simulink model "singleRotor_speedCTRL_dynInflow_PittPeters"  (R2022b)
settings: Solver=ode45  StartTime=0.0  StopTime=55  RelTol=1e-4  EnableMultiTasking=on
InitFcn:
  | dir = pwd; %model directory
  | 
  | %go to look up tables
  | cd('../Look Up Tables/') %look up table directory
  | 
  | % %Ct, Cp, and theta of rotor from BEMT (for comparison)
  | load("BEMT-3.mat");
  | 
  | %Rotor and Pitt-Peters model parameters (M,L,k)
  | load("PP-2.mat");
  | k = model.k; %mass flow correction
  | 
  | %go back to model directory
  | cd(pwd);
  | 
  | %Hide scope plots
  | HidHandles = get(0,'ShowHiddenHandles');
  | set(0,'ShowHiddenHandles','On');
  | AllScopeHandles = findobj(0,'Type','Figure','Tag','SIMULINK_SIMSCOPE_FIGURE');
  | close(AllScopeHandles);
  | set(0,'ShowHiddenHandles',HidHandles);
  | 
  | %Working Directory
  | directory = pwd;
  | 
  | %Atmospheric Properties
  | rho_air = 1.225;  % air density in kg/m^3
  | mu = 1.803e-5; % dynamic viscosity [N-s/m^2]
  | 
  | Vbus = 300;  % Actual bus voltage (volts) that will be applied
  | % Emrax 208
  | R = .0122;  %  resistance, ohms, line-line at room temp
  | L = 125*10^-6;  %  inductance line-line at commutation frequency, henries
  | t_elec = L/R;
  | 
  | Irotor = 256/100^2;  %  kg*m^2 -- From Emrax data sheet
  | Kt_motor = .8005;  %  N*m/Arms (measured from 05/25/2023 test_c data)
  | Ke_motor = .0487*sqrt(2)*60/(2*pi);  %  Vpk/rad/sec
  | Ke = .0487*sqrt(2)*60/(2*pi);   %radians/sec
  | 
  | CurrentSenseMax = 250;  %  Max current sense from controller code
  | BASE_CURRENT = 125;   %  Max current in amps corresponding to normalized control loop current = 1
  | LOOP_FREQUENCY = 35;     % orig: 35 in kHz
  | T_LOOP = .001/LOOP_FREQUENCY;
  | pwm_loop_prescalar = 1;  %Presacalar how many PWM cycles for one current loop execution
  | T_PWM = T_LOOP/pwm_loop_prescalar;  %  Current loop prescaler on PWM is 1 for Uber
  | POLES = 20;
  | BASE_FREQ = 1200; %POLES/2*1300/60;  %  1300 rpm
  | BaseSpeed     = BASE_FREQ*(60.0/(POLES/2.0));
  | 
  | % current loop
  | alpha = 250*2*pi;         % current loop bandwidth
  | 
  | omega = 0;               % omega for de-coupling integrator
  | 
  | % no-load current fit (i0 = a1*omega^2 + a2) [Apk]
  | i_a1 = 8.98e-5;
  | i_a2 = 2.51;
  | 
  | % Current loop
  | %          Motor_Params.ILOOP_BW = (2*PI*1000.0);
  | %        Motor_Params.id_KP = Motor_Params.ILOOP_BW*Motor_Params.StatorInductance;
  | %      Motor_Params.id_KI = Motor_Params.ILOOP_BW*Motor_Params.StatorResistance;
  | %      Motor_Params.iq_KP = Motor_Params.ILOOP_BW*Motor_Params.StatorInductance;
  | %     Motor_Params.iq_KI = Motor_Params.ILOOP_BW*Motor_Params.StatorResistance;
  | I_Kp = alpha*L*1;
  | I_Ki = alpha*R/I_Kp*T_LOOP;
  | %I_Ki = alpha*R*0;
  | 
  | % Speed loop
  | %------------%
  | %NOTES
  | %Originial Kp = 3.0 and Ki = 0.15*Tspeedloop*1.5
  | %Kp = 4.75 and Ki = 2.5e-4 led to only ~1-2s response time indep. of slew rate
  | %Kp = 15 and Ki = 2.1*Tspeedloop*1.5 led to 0.4s response time with slight overshoot
  | %------------%
  | SpeedLoopPrescale = 5;
  | Tspeedloop = T_LOOP*SpeedLoopPrescale;
  | % PID_spd_Kp = 18;   % From Uber code (ORIGINIAL: 3)
  | % PID_spd_Ki = 1*Tspeedloop;   % From Uber code (ORIGINAL: 0.15*Tspeedloop*2)
  | PID_spd_Kp = 31;   % From Uber code (ORIGINIAL: 3)
  | PID_spd_Ki = .128*Tspeedloop;   % From Uber code (ORIGINAL: 0.15*Tspeedloop*2)
  | 
  | Ramp_sec = 1250;    %  Ramp slew rate limiter, [rpm/s]
  | 
  | % Position loop
  | speedErrorPEngage = .003; % Speed error max for position loop to enable
  | % Code has .001 for PEngage, trying something diff here
  | PID_pos_Kp = 3.5; %on MC40: 2.5 (changed on 23 OCT 2021)
  | PID_pos_Ki = .00001; % orig: 0.00003
  | PID_pos_Kd = 8000; % on MC40: 8000
  | 
  | PID_pos_error_sat = .3;  % ORIG = 0.3 Maximum error saturated into position PID (in simulink, not C right now)
  | PID_pos_sat = .25;  %  From code, based on DC bus limit (orig: .25)
  | PID_pos_C1 = .999; % ORIG = 1 Position loop D bandlimit filter
  | PID_pos_C2 = .001;  % ORIG = 0 Position loop D bandlimit filter
  | 
  | 
  | % transfer function of speed estimator is K1*K3*z/(z-K2)
  | %  Pole is at z = K2
  | % z = exp(-sT)
  | f_estpole = 35000;  %orig: 35000
  | K1 = 1/(BASE_FREQ*T_LOOP);   %  Divide by base freq to convert from elec delta-normalized-angle/cycle to [0,1] normalized speed
  |      %  K1 converts delta angle estimate over a loop period to a [0,1] speed estimate
  | K2 = exp(-f_estpole*2*pi*T_LOOP);
  | K3 = 1 - K2;  % Set to make filter have unity gain at 0 frequency (z = 1)
  | 
  | %Rotor properties
  | %{---------------- COAX ------------------------
  | % d_prop = 2.216;   %  diameter propeller [m] 2.032 (coax) 2.216 (stacked)
  | % R_c = d_prop/2*.19; % root cutout [m]
  | % c = 0.08; %chord [m]
  | % nb = 2; %number of blades
  | % sigma = nb*c/pi/(d_prop/2);
  | % I_emp = rotor_params.I_rotor; %from dynamic RPM testing (230313 test k and l)
  | % I_emp = 0.248; %CAD inertia
  | % I_emp = 0.40481; %from dynamic RPM testing (230313 test k and l)
  | % GR = 1.2;
  | % kappa = rotor_params.kappa;
  | % dr = rotor_params.dr;
  | % Cp0 = 5.908e-5; %profile power coefficient (230314 steady)
  | % Cp0 = 6.167e-05; %profile power (230525_test_c steady -- stacked rotor)
  | %-------------------------------------------------
  | %}
  | 
  | %{---------------- UBER ------------------------
  | d_prop = 2*rotor_params.R;   %  diameter propeller [m] 2.032 (coax) 2.216 (stacked)
  | R_c = rotor_params.R_cutout; % root cutout [m]
  | c = rotor_params.c; %chord [m]
  | nb = rotor_params.Nb; %number of blades
  | sigma = nb*c/pi/(d_prop/2);
  | I_emp = rotor_params.I_rotor; %from dynamic RPM testing (230525 test a) [kg*m2]
  | I_m = 0.2717; %from dynamic RPM testing (230525 test a) [kg*m2]
  | % I_m = 2*0.3662; %4-bladed comparison motor inerita. 2X the motor inertia from 231113 testing
  | GR = 1.2;
  | kappa = rotor_params.kappa;
  | dr = rotor_params.dr;
  | Cp0 = rotor_params.Cp0; %profile power (230525_test_c steady -- stacked rotor)
  | %-------------------------------------------------
  | %}
  | 
  | 
  | InitialRPM = 950*GR;
  | omegamech = InitialRPM/60*2*pi;  %  Used to preload Q current voltage integrator
  | 
  | % Serial Message frequency (messages per second)
  | MsgFreq = 1000;
  | 
  | cd(dir);
values from neighbouring files (symbols this model uses):
  Ct = [0 8.42066058624e-05 0.000168413211725 0.000252619817587 0.000348569118235 0.000435711397794 0.000522853677352 0.000609995956911 0.00069713823647 0.000784280516029 0.000871422795587 0.000958565075146 ... (150 elements, 1x150)]    [BEMT-1.mat]    (also in BEMT-2.mat = [-0.000241284312952 -0.00019885713846 -0.000156429963968 -0.; BEMT-3.mat = [-0.000252881464423 -0.00020500571035 -0.00015767832519 -0.0; BEMT-PF-Isolated-1.mat = [-0.000124730397385 6.78902114512e-07 0.000152796242494 0.00; BEMT-PF-Isolated-2.mat = [-0.000124743531158 6.68801957239e-07 0.000152879013625 0.00)
  model =     [DynInflow-1.mat]    (also in PP-1.mat; PP-2.mat; PP-3.mat)
  rotor_params =     [DynInflow-1.mat]    (also in PP-1.mat; PP-2.mat; PP-3.mat)
  theta = [-1.24244156171 -0.730247869575 -0.489791195362 -0.291308360013 -0.0904887039498 0.0775201787218 0.236938510902 0.389966557012 0.537998944025 0.680941129328 0.820002111662 0.955737387113 ... (150 elements, 1x150)]    [BEMT-1.mat]    (also in BEMT-2.mat = [-2.67472972391 -2.52181622329 -2.35655527709 -2.17339529035; BEMT-3.mat = [-2.61565298703 -2.45920727031 -2.29202818901 -2.11251263407; BEMT-PF-Isolated-1.mat = [-2 -1 0 1 2 3 4 5 6 7 8 9 ... (16 elements, 1x16)]; BEMT-PF-Isolated-2.mat = [-2 -1 0 1 2 3 4 5 6 7 8 9 ... (16 elements, 1x16)])
undefined symbols (not defined in the file or in its folder): DiscIntNeverNeededParam
libraries: eeGeneralControl x1
settings Model: ModifiedHistory=4/7/2020 Adding in voltage saturation to mag 1 before SVGEN  Creator=mricci  LastModifiedBy=msa2925
settings SolverCC: AlgebraicLoopSolver=TrustRegion
settings DataIOCC: LimitDataPoints=on  SaveFormat=Array  SignalLoggingSaveFormat=ModelDataLogs  ReturnWorkspaceOutputs=off
settings OptimizationCC: ExpressionDepthLimit=2147483647  InitFltsAndDblsToZero=on  LifeSpan=inf
settings DebuggingCC: UnderspecifiedInitializationDetection=Classic  MergeDetectMultiDrivingBlocksExec=none  SolverPrmCheckMsg=warning  FcnCallInpInsideContextMsg=warning  UnconnectedInputMsg=warning  UnconnectedOutputMsg=warning  UnconnectedLineMsg=warning  StateNameClashWarn=warning  SFUnexpectedBacktrackingDiag=warning  SFNoUnconditionalDefaultTransitionDiag=warning  SFExecutionAtInitializationDiag=none  SFMachineParentedDataDiag=warning  ArithmeticOperatorsInVariantConditions=warning
settings HardwareCC: ProdBitPerPointer=32  ProdBitPerSizeT=32  ProdBitPerPtrDiffT=32  ProdLargestAtomicFloat=None  ProdIntDivRoundTo=Undefined  ProdEndianess=Unspecified  ProdWordSize=32  ProdHWDeviceType=32-bit Generic
settings ModelReferenceCC: EnableRefExpFcnMdlSchedulingChecks=on  PropagateSignalLabelsOutOfModel=off
settings RTWCC: DLArmComputeVersion=19.05
settings CodeAppCC: StateflowObjectComments=on
settings GRTTargetCC: TargetLangStandard=C89/C90 (ANSI)  CombineOutputUpdateFcns=off  GRTInterface=on
settings ConfigComp: CovMetricSettings=dw  CovSaveCumulativeToWorkspaceVar=on  CovSaveSingleToWorkspaceVar=on

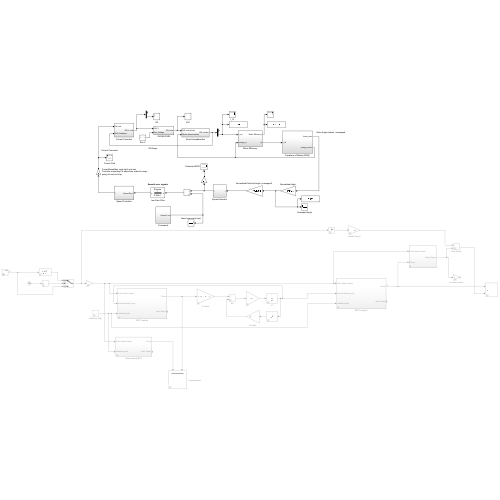
[thumbnail: Simulink's stored preview of the top-level diagram]
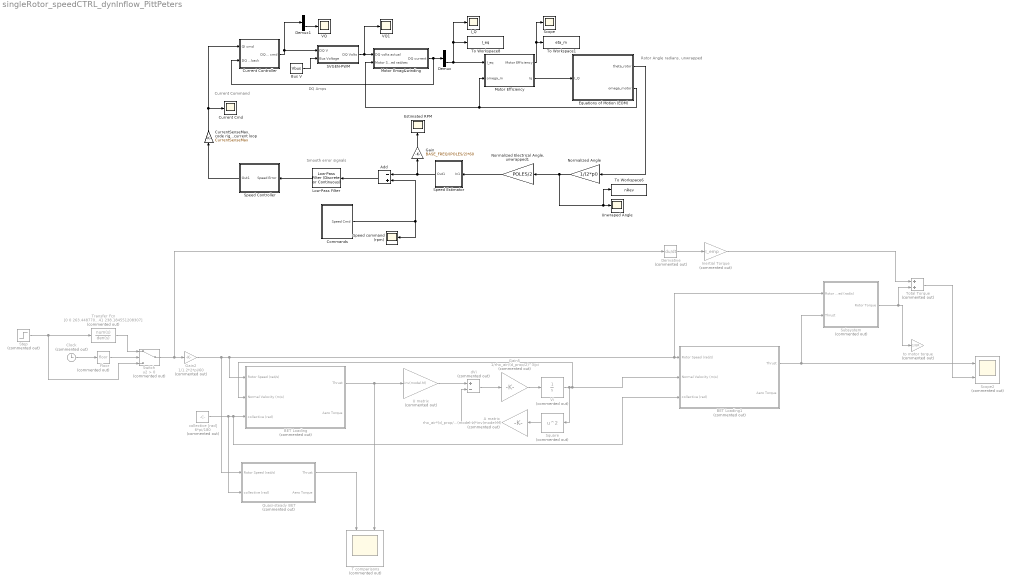
== system singleRotor_speedCTRL_dynInflow_PittPeters ==
  note: Smooth error signals
  note: Current Command
  note: Rotor Angle radians, unwrapped
  note: DQ Amps
  A matrix : Gain  Commented=on  Gain=rho_air*(d_prop/2)^2*pi*k*inv(model.L)*inv(model.M)
  Add : Sum  Inputs=-+
  BET Loading : Subsystem  Commented=on
  BET Loading1 : Subsystem  Commented=on
  Bus V : Constant  Value=Vbus
  Clock : Clock  Commented=on
  Commands : Subsystem
  Current Cmd : Scope
  Current Controller : Subsystem
  "CurrentSenseMax, code right now has Controller outputting PU amps then scaled to amps going into current loop" : Gain  Gain=CurrentSenseMax
  Demux : Demux  Outputs=2
  Demux1 : Demux  Outputs=2
  Derivative : Derivative  Commented=on
  Equations of Motion (EOM) : Subsystem
  Estimated RPM : Scope
  Floor : Rounding  Commented=on
  Gain : Gain  Gain=BASE_FREQ/(POLES/2)*60
  Gain2 : Gain  Commented=on  Gain=1/1.2*2*pi/60
  Gain5 : Gain  Commented=on  Gain=1/rho_air/(d_prop/2)^3/pi
  I_Q : Scope
  Inertial Torque : Gain  Commented=on  Gain=I_emp
  Low-Pass Filter : eeGeneralControl/Low-Pass Filter (Discrete or Continuous)  K=1  T=3e-2  B=inf  A=-inf  init_option=Inherited from block input  x0=0  Ts=-1
  Motor Efficiency : Subsystem
  Motor Emag&winding : Subsystem
  Normalized Angle : Gain  Gain=1/(2*pi)
  "Normalized Electrical Angle, unwrapped1" : Gain  Gain=POLES/2
  Quasi-steady BET : Subsystem  Commented=on
  SVGEN-PWM : Subsystem
  Scope : Scope
  Scope2 : Scope  Commented=on  NumInputPorts=2
  Speed Controller : Subsystem
  Speed Estimator : Subsystem
  Speed command (rpm) : Scope
  Square : Math  Commented=on  Operator=square
  Step : Step  Commented=on  Time=50  Before=InitialRPM  After=InitialRPM+30*GR  SampleTime=0
  Subsystem : Subsystem  Commented=on
  Switch : Switch  Commented=on  Criteria=u2 > Threshold  SaturateOnIntegerOverflow=off  InputSameDT=off
  T comparisons : Scope  Commented=on  NumInputPorts=2
  To Workspace1 : ToWorkspace  VariableName=eta_m  SaveFormat=Timeseries  SampleTime=-1
  To Workspace6 : ToWorkspace  VariableName=nRev  SaveFormat=Timeseries  SampleTime=-1
  To Workspace8 : ToWorkspace  VariableName=I_eq  SaveFormat=Timeseries  SampleTime=-1
  Total Torque : Sum  Commented=on
  Transfer Fcn : TransferFcn  Commented=on  Numerator="[0\t0\t263.448770344578]"  Denominator="[1\t17.1002833911441\t238.184551208307]"
  U matrix : Gain  Commented=on  Gain=inv(model.M)
  Unwraped Angle : Scope
  VQ : Scope
  VQ1 : Scope
  Vi : Integrator  Commented=on  InitialCondition=5.9
  collective [rad] : Constant  Commented=on  Value=6*pi/180
  dVi : Sum  Commented=on  Inputs=+-
  to motor torque : Gain  Commented=on  Gain=1/GR
  wires:
  Speed Estimator/1(Out1) -> Add/1, Gain/1
  Gain/1 -> Estimated RPM/1
  Add/1 -> Low-Pass Filter/1
  "CurrentSenseMax, code right now has Controller outputting PU amps then scaled to amps going into current loop"/1 -> Current Controller/1(QI cmd), Current Cmd/1
  Equations of Motion (EOM)/2(omega_motor) -> Motor Efficiency/2(omega_m), Motor Emag&winding/2(Motor Speed rad/sec)
  Motor Emag&winding/1(DQ current) -> Current Controller/2(DQ I feedback), Demux/1
  Demux/2 -> Motor Efficiency/1(I_eq), To Workspace8/1, I_Q/1
  Equations of Motion (EOM)/1(theta_rotor) -> Normalized Angle/1
  Normalized Angle/1 -> "Normalized Electrical Angle, unwrapped1"/1, To Workspace6/1, Unwraped Angle/1
  "Normalized Electrical Angle, unwrapped1"/1 -> Speed Estimator/1(In1)
  Commands/1(Speed Cmd) -> Add/2, Speed command (rpm)/1
  Speed Controller/1(Out1) -> "CurrentSenseMax, code right now has Controller outputting PU amps then scaled to amps going into current loop"/1
  Demux1/2 -> VQ/1
  Low-Pass Filter/1 -> Speed Controller/1(Speed Error)
  SVGEN-PWM/1(DQ Volts) -> VQ1/1, Motor Emag&winding/1(DQ volts actual)
  Bus V/1 -> SVGEN-PWM/2(Bus Voltage)
  Current Controller/1(DQ V cmd) -> SVGEN-PWM/1(DQ V), Demux1/1
  Motor Efficiency/2(Iq) -> Equations of Motion (EOM)/1(I_Q)
  Motor Efficiency/1(Motor Efficiency) -> Scope/1, To Workspace1/1
  Gain2/1 -> Subsystem/1(Rotor Speed (rad/s)), BET Loading1/1(Rotor Speed (rad/s)), BET Loading/1(Rotor Speed (rad/s)), Quasi-steady BET/1(Rotor Speed (rad/s))
  A matrix/1 -> dVi/2
  Quasi-steady BET/1(Thrust) -> T comparisons/2
  collective [rad]/1 -> BET Loading/3(collective (rad)), BET Loading1/3(collective (rad)), Quasi-steady BET/2(collective (rad))
  Square/1 -> A matrix/1
  U matrix/1 -> dVi/1
  Gain5/1 -> Vi/1
  BET Loading/1(Thrust) -> T comparisons/1, U matrix/1
  dVi/1 -> Gain5/1
  Vi/1 -> BET Loading1/2(Normal Velocity (m/s)), BET Loading/2(Normal Velocity (m/s)), Square/1
  BET Loading1/1(Thrust) -> Subsystem/2(Thrust), Scope2/1
  Switch/1 -> Derivative/1, Gain2/1
  Transfer Fcn/1 -> Switch/1
  Step/1 -> Transfer Fcn/1, Switch/3
  Floor/1 -> Switch/2
  Clock/1 -> Floor/1
  Subsystem/1(Rotor Torque) -> Total Torque/2, to motor torque/1
  Derivative/1 -> Inertial Torque/1
  Total Torque/1 -> Scope2/2
  Inertial Torque/1 -> Total Torque/1

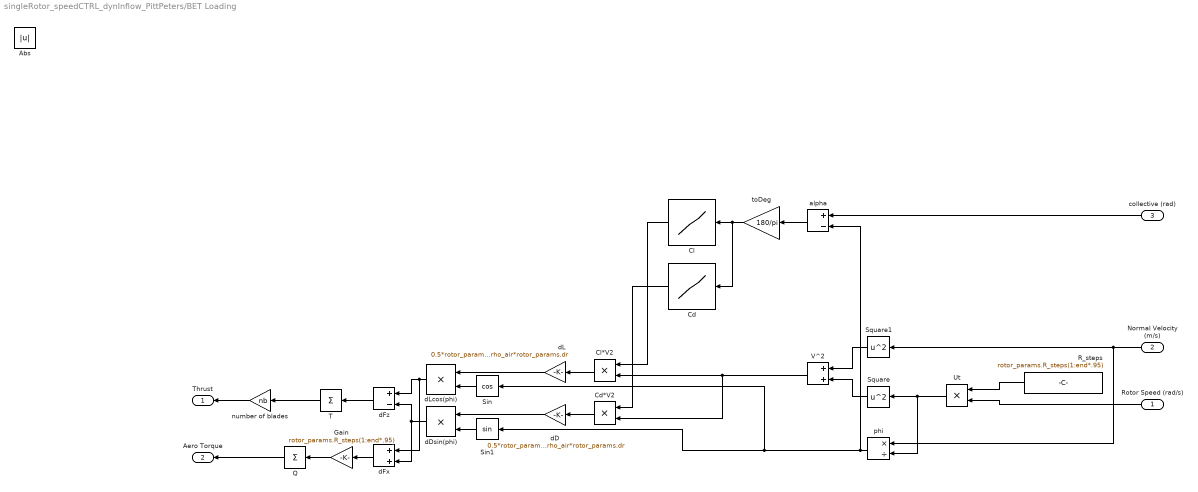
== system singleRotor_speedCTRL_dynInflow_PittPeters/BET Loading ==
  Rotor Speed (rad/s) : Inport
  Normal Velocity (m/s) : Inport  Port=2
  collective (rad) : Inport  Port=3
  Abs : Abs  SaturateOnIntegerOverflow=off
  Cd : Lookup_n-D  NumberOfTableDimensions=1  BreakpointsForDimension1=rotor_params.AoA  BreakpointsForDimension2=[1:3]  Table=rotor_params.Cd  InternalRulePriority=Speed  RndMeth=Simplest
  Cd*V2 : Product
  Cl : Lookup_n-D  NumberOfTableDimensions=1  BreakpointsForDimension1=rotor_params.AoA  BreakpointsForDimension2=[1:3]  Table=rotor_params.Cl  UseLastTableValue=on  InternalRulePriority=Speed  RndMeth=Simplest
  Cl*V2 : Product
  Gain : Gain  Gain=rotor_params.R_steps(1:end*.95)
  Q : Sum  Inputs=+
  R_steps : Constant  Value=rotor_params.R_steps(1:end*.95)
  Sin : Trigonometry  Operator=cos
  Sin1 : Trigonometry
  Square : Math  Operator=square
  Square1 : Math  Operator=square
  T : Sum  Inputs=+
  Ut : Product
  V^2 : Sum
  alpha : Sum  Inputs=+-
  dD : Gain  Gain=0.5*rotor_params.c*rho_air*rotor_params.dr
  dDsin(phi) : Product
  dFx : Sum
  dFz : Sum  Inputs=+-
  dL : Gain  Gain=0.5*rotor_params.c*rho_air*rotor_params.dr
  dLcos(phi) : Product
  number of blades : Gain  Gain=nb
  phi : Product  Inputs=*/
  toDeg : Gain  Gain=180/pi
  Thrust : Outport
  Aero Torque : Outport  Port=2
  wires:
  T/1 -> number of blades/1
  alpha/1 -> toDeg/1
  Normal Velocity (m/s)/1 -> phi/1, Square1/1
  Rotor Speed (rad/s)/1 -> Ut/2
  phi/1 -> Sin/1, Sin1/1, alpha/2
  collective (rad)/1 -> alpha/1
  Square/1 -> V^2/2
  Square1/1 -> V^2/1
  Ut/1 -> phi/2, Square/1
  V^2/1 -> Cl*V2/2, Cd*V2/2
  R_steps/1 -> Ut/1
  Cl*V2/1 -> dL/1
  Cd*V2/1 -> dD/1
  Sin/1 -> dLcos(phi)/2
  dL/1 -> dLcos(phi)/1
  dD/1 -> dDsin(phi)/1
  Sin1/1 -> dDsin(phi)/2
  dLcos(phi)/1 -> dFx/1, dFz/1
  dDsin(phi)/1 -> dFx/2, dFz/2
  dFz/1 -> T/1
  number of blades/1 -> Thrust/1
  toDeg/1 -> Cl/1, Cd/1
  Cd/1 -> Cd*V2/1
  Q/1 -> Aero Torque/1
  dFx/1 -> Gain/1
  Gain/1 -> Q/1
  Cl/1 -> Cl*V2/1

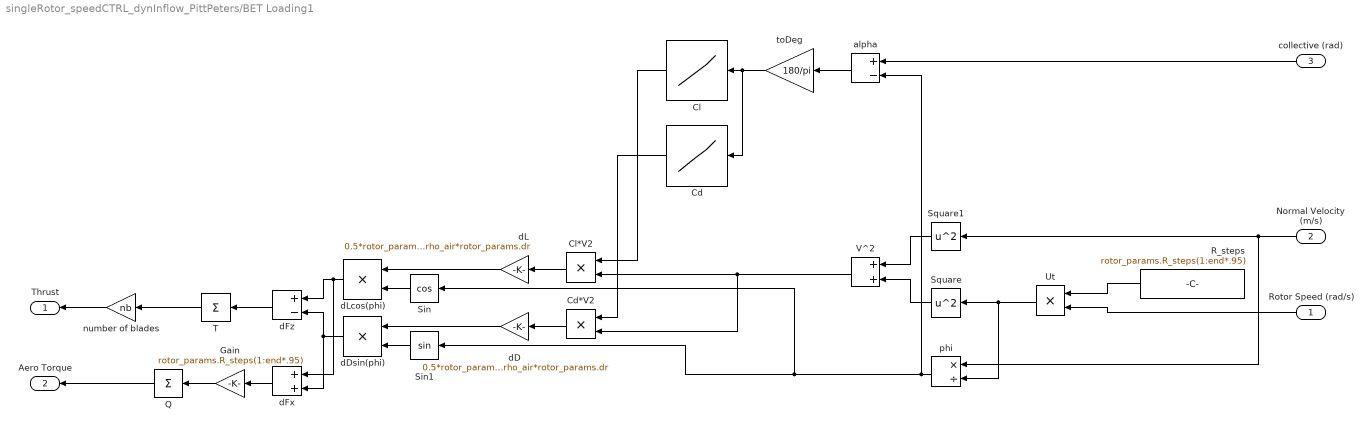
== system singleRotor_speedCTRL_dynInflow_PittPeters/BET Loading1 ==
  Rotor Speed (rad/s) : Inport
  Normal Velocity (m/s) : Inport  Port=2
  collective (rad) : Inport  Port=3
  Cd : Lookup_n-D  NumberOfTableDimensions=1  BreakpointsForDimension1=rotor_params.AoA  BreakpointsForDimension2=[1:3]  Table=rotor_params.Cd  InternalRulePriority=Speed  RndMeth=Simplest
  Cd*V2 : Product
  Cl : Lookup_n-D  NumberOfTableDimensions=1  BreakpointsForDimension1=rotor_params.AoA  BreakpointsForDimension2=[1:3]  Table=rotor_params.Cl  UseLastTableValue=on  InternalRulePriority=Speed  RndMeth=Simplest
  Cl*V2 : Product
  Gain : Gain  Gain=rotor_params.R_steps(1:end*.95)
  Q : Sum  Inputs=+
  R_steps : Constant  Value=rotor_params.R_steps(1:end*.95)
  Sin : Trigonometry  Operator=cos
  Sin1 : Trigonometry
  Square : Math  Operator=square
  Square1 : Math  Operator=square
  T : Sum  Inputs=+
  Ut : Product
  V^2 : Sum
  alpha : Sum  Inputs=+-
  dD : Gain  Gain=0.5*rotor_params.c*rho_air*rotor_params.dr
  dDsin(phi) : Product
  dFx : Sum
  dFz : Sum  Inputs=+-
  dL : Gain  Gain=0.5*rotor_params.c*rho_air*rotor_params.dr
  dLcos(phi) : Product
  number of blades : Gain  Gain=nb
  phi : Product  Inputs=*/
  toDeg : Gain  Gain=180/pi
  Thrust : Outport
  Aero Torque : Outport  Port=2
  wires:
  T/1 -> number of blades/1
  alpha/1 -> toDeg/1
  Normal Velocity (m/s)/1 -> phi/1, Square1/1
  Rotor Speed (rad/s)/1 -> Ut/2
  phi/1 -> Sin/1, Sin1/1, alpha/2
  collective (rad)/1 -> alpha/1
  Square/1 -> V^2/2
  Square1/1 -> V^2/1
  Ut/1 -> phi/2, Square/1
  V^2/1 -> Cl*V2/2, Cd*V2/2
  R_steps/1 -> Ut/1
  Cl*V2/1 -> dL/1
  Cd*V2/1 -> dD/1
  Sin/1 -> dLcos(phi)/2
  dL/1 -> dLcos(phi)/1
  dD/1 -> dDsin(phi)/1
  Sin1/1 -> dDsin(phi)/2
  dLcos(phi)/1 -> dFx/1, dFz/1
  dDsin(phi)/1 -> dFx/2, dFz/2
  dFz/1 -> T/1
  number of blades/1 -> Thrust/1
  toDeg/1 -> Cd/1, Cl/1
  Cd/1 -> Cd*V2/1
  Q/1 -> Aero Torque/1
  dFx/1 -> Gain/1
  Gain/1 -> Q/1
  Cl/1 -> Cl*V2/1

== system singleRotor_speedCTRL_dynInflow_PittPeters/Commands ==
  "Normalized Speed [0,1] relative to \"base freq" : Gain  Gain=1/BaseSpeed
  Rate Limiter : RateLimiter  RisingSlewLimit=Ramp_sec  FallingSlewLimit=-Ramp_sec  SampleTimeMode=inherited  InitialCondition=InitialRPM/BaseSpeed
  Step : Step  Time=50  Before=InitialRPM  After=InitialRPM + 30*GR  SampleTime=0
  To Workspace5 : ToWorkspace  VariableName=Speed_cmd  SaveFormat=Timeseries  SampleTime=-1
  td : TransportDelay  DelayTime=.02
  Speed Cmd : Outport
  wires:
  "Normalized Speed [0,1] relative to \"base freq"/1 -> Speed Cmd/1
  Step/1 -> td/1, To Workspace5/1
  td/1 -> "Normalized Speed [0,1] relative to \"base freq"/1

== system singleRotor_speedCTRL_dynInflow_PittPeters/Current Controller ==
  note: Q current PI controller
  note: D current PI controller
  note: D Current Reference
  note: D Current Feedback
  note: Q Current Reference
  note: Discrete
      | time control
      | law
  QI cmd : Inport
  DQ I feedback : Inport  Port=2
  1/Ts gain DT integrator : DiscreteIntegrator  gainval=1/T_LOOP  InitialCondition=80  SampleTime=-1  LimitOutput=on  UpperSaturationLimit=Vbus*sqrt(3)  LowerSaturationLimit=-Vbus*sqrt(3)  ICPrevOutput=DiscIntNeverNeededParam  ICPrevScaledInput=DiscIntNeverNeededParam
  Constant : Constant  Value=0
  Demux : Demux  Outputs=2
  Gain : Gain  Gain=I_Kp
  Gain1 : Gain  Gain=I_Ki
  Gain2 : Gain  Gain=I_Kp
  Gain3 : Gain  Gain=I_Ki
  K=1/Ts DT itegrator : DiscreteIntegrator  gainval=1/T_LOOP  InitialCondition=-2  SampleTime=-1  LimitOutput=on  UpperSaturationLimit=Vbus*sqrt(3)  LowerSaturationLimit=-Vbus*sqrt(3)  ICPrevOutput=DiscIntNeverNeededParam  ICPrevScaledInput=DiscIntNeverNeededParam
  Mux1 : Mux  Inputs=2
  Sum : Sum  Inputs=|++
  Sum1 : Sum  Inputs=|++
  Sum2 : Sum  Inputs=|+-
  Sum3 : Sum  Inputs=|+-
  DQ V cmd : Outport
  wires:
  Mux1/1 -> DQ V cmd/1
  Constant/1 -> Sum2/1
  QI cmd/1 -> Sum3/1
  Sum/1 -> Mux1/1
  Sum1/1 -> Mux1/2
  DQ I feedback/1 -> Demux/1
  Demux/1 -> Sum2/2
  Demux/2 -> Sum3/2
  K=1/Ts DT itegrator/1 -> Sum/2
  Gain1/1 -> K=1/Ts DT itegrator/1
  Gain/1 -> Sum/1, Gain1/1
  Sum2/1 -> Gain/1
  Sum3/1 -> Gain2/1
  Gain2/1 -> Sum1/1, Gain3/1
  Gain3/1 -> 1/Ts gain DT integrator/1
  1/Ts gain DT integrator/1 -> Sum1/2

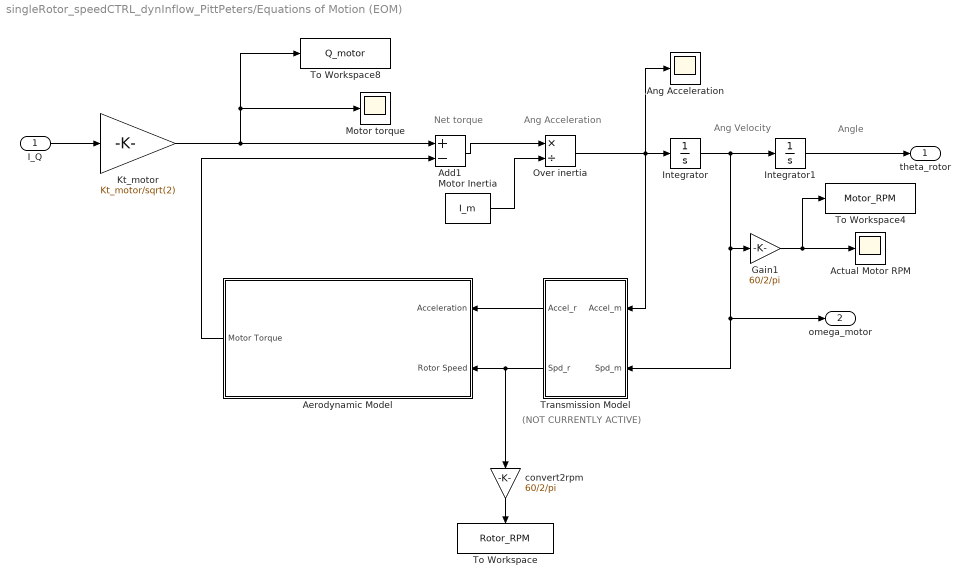
== system singleRotor_speedCTRL_dynInflow_PittPeters/Equations of Motion (EOM) ==
  note: (NOT CURRENTLY ACTIVE)
  note: Ang Acceleration
  note: Angle
  note: Ang Velocity
  note: Net torque
  I_Q : Inport
  Actual Motor RPM : Scope
  Add1 : Sum  Inputs=+-
  Aerodynamic Model : Subsystem
  Ang Acceleration : Scope
  Gain1 : Gain  Gain=60/2/pi
  Integrator : Integrator  InitialCondition=InitialRPM*2*pi/60
  Integrator1 : Integrator
  Kt_motor : Gain  Gain=Kt_motor/sqrt(2)
  Motor Inertia : Constant  Value=I_m
  Motor torque : Scope
  Over inertia : Product  Inputs=*/
  To Workspace : ToWorkspace  VariableName=Rotor_RPM  SaveFormat=Timeseries  SampleTime=-1
  To Workspace4 : ToWorkspace  VariableName=Motor_RPM  SaveFormat=Timeseries  SampleTime=-1
  To Workspace8 : ToWorkspace  VariableName=Q_motor  SaveFormat=Timeseries  SampleTime=-1
  Transmission Model : Subsystem
  convert2rpm : Gain  Gain=60/2/pi
  theta_rotor : Outport
  omega_motor : Outport  Port=2
  wires:
  I_Q/1 -> Kt_motor/1
  Integrator1/1 -> theta_rotor/1
  Add1/1 -> Over inertia/1
  Kt_motor/1 -> To Workspace8/1, Motor torque/1, Add1/1
  Gain1/1 -> To Workspace4/1, Actual Motor RPM/1
  Aerodynamic Model/1(Motor Torque) -> Add1/2
  Motor Inertia/1 -> Over inertia/2
  convert2rpm/1 -> To Workspace/1
  Integrator/1 -> Integrator1/1, Transmission Model/2(Spd_m), omega_motor/1, Gain1/1
  Over inertia/1 -> Integrator/1, Transmission Model/1(Accel_m), Ang Acceleration/1
  Transmission Model/2(Spd_r) -> Aerodynamic Model/2(Rotor Speed), convert2rpm/1
  Transmission Model/1(Accel_r) -> Aerodynamic Model/1(Acceleration)

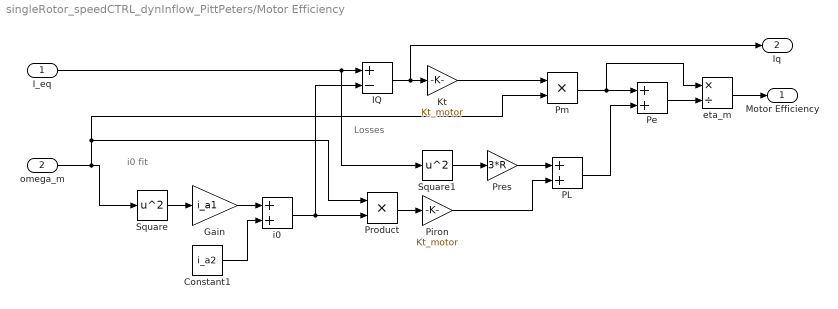
== system singleRotor_speedCTRL_dynInflow_PittPeters/Motor Efficiency ==
  note: Losses
  note: i0 fit
  I_eq : Inport
  omega_m : Inport  Port=2
  Constant1 : Constant  Value=i_a2
  Gain : Gain  Gain=i_a1
  IQ : Sum  Inputs=+-
  Kt : Gain  Gain=Kt_motor
  PL : Sum
  Pe : Sum
  Piron : Gain  Gain=Kt_motor
  Pm : Product
  Pres : Gain  Gain=3*R
  Product : Product
  Square : Math  Operator=square
  Square1 : Math  Operator=square
  eta_m : Product  Inputs=*/
  i0 : Sum
  Motor Efficiency : Outport
  Iq : Outport  Port=2
  wires:
  IQ/1 -> Iq/1, Kt/1
  Kt/1 -> Pm/1
  Pm/1 -> eta_m/1, Pe/1
  Pe/1 -> eta_m/2
  eta_m/1 -> Motor Efficiency/1
  Gain/1 -> i0/1
  Constant1/1 -> i0/2
  Square/1 -> Gain/1
  PL/1 -> Pe/2
  Pres/1 -> PL/1
  I_eq/1 -> Square1/1, IQ/1
  Square1/1 -> Pres/1
  omega_m/1 -> Product/1, Pm/2, Square/1
  Product/1 -> Piron/1
  Piron/1 -> PL/2
  i0/1 -> Product/2, IQ/2

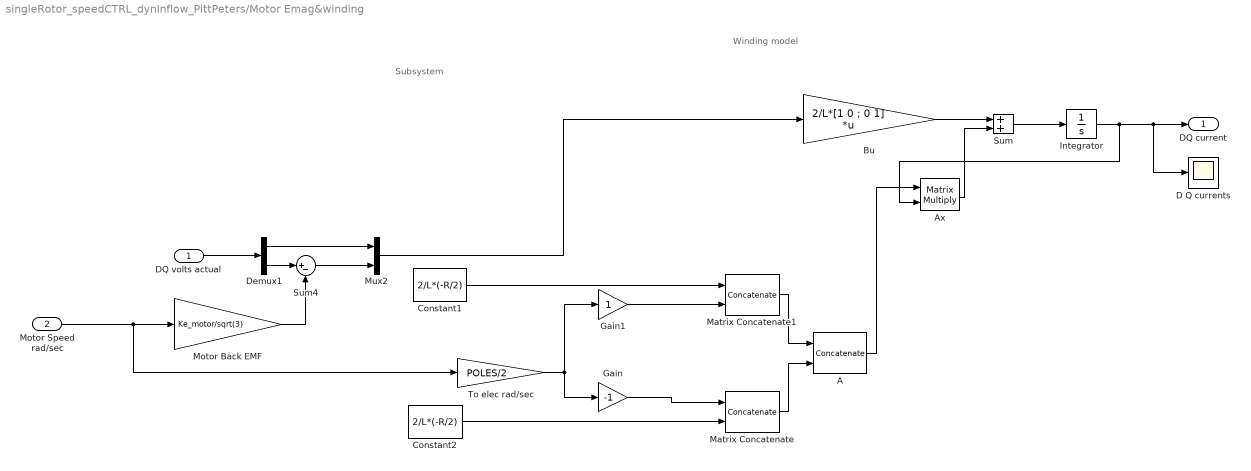
== system singleRotor_speedCTRL_dynInflow_PittPeters/Motor Emag&winding ==
  note: Subsystem
  note: Winding model
  DQ volts actual : Inport
  Motor Speed rad/sec : Inport  Port=2
  A : Concatenate  Mode=Multidimensional array
  Ax : Product  Multiplication=Matrix(*)  RndMeth=Zero
  Bu : Gain  Gain=2/L*[1 0 ; 0 1]  Multiplication=Matrix(K*u)
  Constant1 : Constant  Value=2/L*(-R/2)
  Constant2 : Constant  Value=2/L*(-R/2)
  D Q currents : Scope
  Demux1 : Demux  Outputs=2
  Gain : Gain  Gain=-1
  Gain1 : Gain
  Integrator : Integrator  InitialCondition=[0 25]
  Matrix Concatenate : Concatenate  Mode=Multidimensional array  ConcatenateDimension=2
  Matrix Concatenate1 : Concatenate  Mode=Multidimensional array  ConcatenateDimension=2
  Motor Back EMF : Gain  Gain=Ke_motor/sqrt(3)
  Mux2 : Mux  Inputs=2
  Sum : Sum
  Sum4 : Sum  Inputs=|+-
  To elec rad/sec : Gain  Gain=POLES/2
  DQ current : Outport
  wires:
  Demux1/1 -> Mux2/1
  Demux1/2 -> Sum4/1
  Sum4/1 -> Mux2/2
  Motor Back EMF/1 -> Sum4/2
  DQ volts actual/1 -> Demux1/1
  Integrator/1 -> DQ current/1, D Q currents/1, Ax/2
  Gain/1 -> Matrix Concatenate/1
  To elec rad/sec/1 -> Gain1/1, Gain/1
  Gain1/1 -> Matrix Concatenate1/2
  Constant2/1 -> Matrix Concatenate/2
  Constant1/1 -> Matrix Concatenate1/1
  Matrix Concatenate/1 -> A/2
  Matrix Concatenate1/1 -> A/1
  A/1 -> Ax/1
  Ax/1 -> Sum/2
  Motor Speed rad/sec/1 -> To elec rad/sec/1, Motor Back EMF/1
  Bu/1 -> Sum/1
  Sum/1 -> Integrator/1
  Mux2/1 -> Bu/1

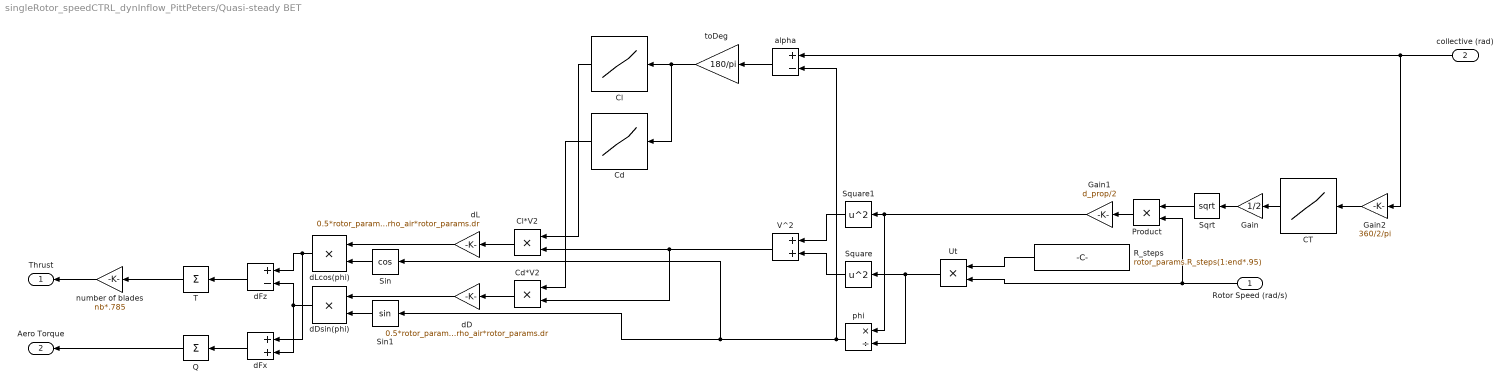
== system singleRotor_speedCTRL_dynInflow_PittPeters/Quasi-steady BET ==
  Rotor Speed (rad/s) : Inport
  collective (rad) : Inport  Port=2
  CT : Lookup_n-D  NumberOfTableDimensions=1  BreakpointsForDimension1=theta  BreakpointsForDimension2=[1:3]  Table=Ct  UseLastTableValue=on  InternalRulePriority=Speed  RndMeth=Simplest
  Cd : Lookup_n-D  NumberOfTableDimensions=1  BreakpointsForDimension1=rotor_params.AoA  BreakpointsForDimension2=[1:3]  Table=rotor_params.Cd  InternalRulePriority=Speed  RndMeth=Simplest
  Cd*V2 : Product
  Cl : Lookup_n-D  NumberOfTableDimensions=1  BreakpointsForDimension1=rotor_params.AoA  BreakpointsForDimension2=[1:3]  Table=rotor_params.Cl  UseLastTableValue=on  InternalRulePriority=Speed  RndMeth=Simplest
  Cl*V2 : Product
  Gain : Gain  Gain=1/2
  Gain1 : Gain  Gain=d_prop/2
  Gain2 : Gain  Gain=360/2/pi
  Product : Product
  Q : Sum  Inputs=+
  R_steps : Constant  Value=rotor_params.R_steps(1:end*.95)
  Sin : Trigonometry  Operator=cos
  Sin1 : Trigonometry
  Sqrt : Sqrt
  Square : Math  Operator=square
  Square1 : Math  Operator=square
  T : Sum  Inputs=+
  Ut : Product
  V^2 : Sum
  alpha : Sum  Inputs=+-
  dD : Gain  Gain=0.5*rotor_params.c*rho_air*rotor_params.dr
  dDsin(phi) : Product
  dFx : Sum
  dFz : Sum  Inputs=+-
  dL : Gain  Gain=0.5*rotor_params.c*rho_air*rotor_params.dr
  dLcos(phi) : Product
  number of blades : Gain  Gain=nb*.785
  phi : Product  Inputs=*/
  toDeg : Gain  Gain=180/pi
  Thrust : Outport
  Aero Torque : Outport  Port=2
  wires:
  T/1 -> number of blades/1
  alpha/1 -> toDeg/1
  Rotor Speed (rad/s)/1 -> Product/2, Ut/2
  phi/1 -> Sin/1, Sin1/1, alpha/2
  collective (rad)/1 -> Gain2/1, alpha/1
  Square/1 -> V^2/2
  Square1/1 -> V^2/1
  Ut/1 -> phi/2, Square/1
  V^2/1 -> Cl*V2/2, Cd*V2/2
  R_steps/1 -> Ut/1
  Cl*V2/1 -> dL/1
  Cd*V2/1 -> dD/1
  Sin/1 -> dLcos(phi)/2
  dL/1 -> dLcos(phi)/1
  dD/1 -> dDsin(phi)/1
  Sin1/1 -> dDsin(phi)/2
  dLcos(phi)/1 -> dFx/1, dFz/1
  dDsin(phi)/1 -> dFx/2, dFz/2
  dFz/1 -> T/1
  number of blades/1 -> Thrust/1
  toDeg/1 -> Cd/1, Cl/1
  Cl/1 -> Cl*V2/1
  Cd/1 -> Cd*V2/1
  dFx/1 -> Q/1
  Q/1 -> Aero Torque/1
  CT/1 -> Gain/1
  Gain/1 -> Sqrt/1
  Sqrt/1 -> Product/1
  Product/1 -> Gain1/1
  Gain2/1 -> CT/1
  Gain1/1 -> phi/1, Square1/1

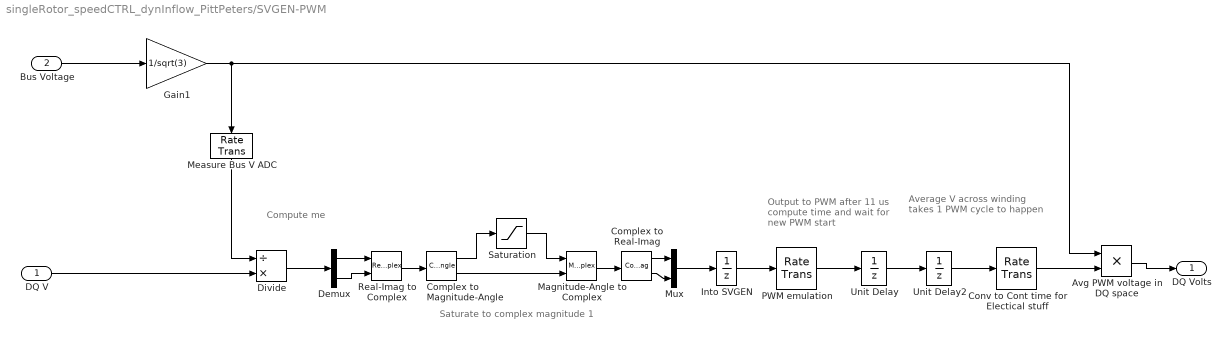
== system singleRotor_speedCTRL_dynInflow_PittPeters/SVGEN-PWM ==
  note: Saturate to complex magnitude 1
  note: Output to PWM
      | after 11 us compute time
      | and wait for new PWM start
  note: Average V
      | across winding
      | takes 1 PWM
      | cycle to happen
  note: Compute
      | me
  DQ V : Inport
  Bus Voltage : Inport  Port=2
  Avg PWM voltage in DQ space : Product  RndMeth=Zero
  Complex to Magnitude-Angle : ComplexToMagnitudeAngle
  Complex to Real-Imag : ComplexToRealImag
  Conv to Cont time for Electical stuff : RateTransition
  Demux : Demux  Outputs=2
  Divide : Product  Inputs=/*
  Gain1 : Gain  Gain=1/sqrt(3)
  Into SVGEN : UnitDelay  InitialCondition=[ 0 ; omegamech*Ke/Vbus]  SampleTime=-1
  Magnitude-Angle to Complex : MagnitudeAngleToComplex
  Measure Bus V ADC : RateTransition  OutPortSampleTime=T_LOOP
  Mux : Mux  Inputs=2
  PWM emulation : RateTransition  OutPortSampleTime=T_PWM
  Real-Imag to Complex : RealImagToComplex
  Saturation : Saturate  UpperLimit=1  LowerLimit=-1
  Unit Delay : UnitDelay  InitialCondition=[ 0 ; omegamech*Ke/Vbus]  SampleTime=-1
  Unit Delay2 : UnitDelay  InitialCondition=[ 0 ; omegamech*Ke/Vbus]  SampleTime=-1
  DQ Volts : Outport
  wires:
  Into SVGEN/1 -> PWM emulation/1
  Unit Delay/1 -> Unit Delay2/1
  PWM emulation/1 -> Unit Delay/1
  Unit Delay2/1 -> Conv to Cont time for Electical stuff/1
  Measure Bus V ADC/1 -> Divide/1
  DQ V/1 -> Divide/2
  Conv to Cont time for Electical stuff/1 -> Avg PWM voltage in DQ space/2
  Avg PWM voltage in DQ space/1 -> DQ Volts/1
  Mux/1 -> Into SVGEN/1
  Divide/1 -> Demux/1
  Demux/1 -> Real-Imag to Complex/1
  Demux/2 -> Real-Imag to Complex/2
  Real-Imag to Complex/1 -> Complex to Magnitude-Angle/1
  Complex to Magnitude-Angle/1 -> Saturation/1
  Saturation/1 -> Magnitude-Angle to Complex/1
  Complex to Magnitude-Angle/2 -> Magnitude-Angle to Complex/2
  Magnitude-Angle to Complex/1 -> Complex to Real-Imag/1
  Complex to Real-Imag/1 -> Mux/1
  Complex to Real-Imag/2 -> Mux/2
  Bus Voltage/1 -> Gain1/1
  Gain1/1 -> Measure Bus V ADC/1, Avg PWM voltage in DQ space/1

== system singleRotor_speedCTRL_dynInflow_PittPeters/Speed Controller ==
  Speed Error : Inport
  1/integraltime to match code since Simulink integrator has Ts term : Gain  Gain=1/(T_LOOP*SpeedLoopPrescale)
  Add1 : Sum
  ControllerIN : Scope
  Discrete-Time Integrator : DiscreteIntegrator  InitialCondition=.03  SampleTime=-1  ICPrevOutput=DiscIntNeverNeededParam  ICPrevScaledInput=DiscIntNeverNeededParam
  Product : Product  RndMeth=Zero
  Product1 : Product  RndMeth=Zero
  Speed I gain : Constant  Value=PID_spd_Ki
  Speed P gain : Constant  Value=PID_spd_Kp
  Out1 : Outport
  wires:
  Speed P gain/1 -> Product1/1
  1/integraltime to match code since Simulink integrator has Ts term/1 -> Discrete-Time Integrator/1
  Product/1 -> 1/integraltime to match code since Simulink integrator has Ts term/1
  Speed I gain/1 -> Product/2
  Add1/1 -> Product1/2
  Product1/1 -> Out1/1
  Discrete-Time Integrator/1 -> Add1/2, ControllerIN/1
  Speed Error/1 -> Add1/1, Product/1

== system singleRotor_speedCTRL_dynInflow_PittPeters/Speed Estimator ==
  note: Speed Estimator
  In1 : Inport
  Add1 : Sum  Inputs=+-
  Add2 : Sum  SampleTime=T_LOOP
  DeltaAngle : Scope
  Filter gain for unity at 0 freq : Gain  Gain=K3
  Sampling : UnitDelay  SampleTime=-1
  Set filer pole : Gain  Gain=K2
  Unit Delay1 : UnitDelay  SampleTime=-1
  Unit Delay2 : UnitDelay  InitialCondition=.021  SampleTime=T_LOOP
  "[0,1] normalization unfiltered speed est from delta angle" : Gain  Gain=K1
  Out1 : Outport
  wires:
  Sampling/1 -> Add1/1, Unit Delay1/1
  Unit Delay1/1 -> Add1/2
  In1/1 -> Sampling/1
  Add2/1 -> Out1/1, Unit Delay2/1
  "[0,1] normalization unfiltered speed est from delta angle"/1 -> Filter gain for unity at 0 freq/1
  Unit Delay2/1 -> Set filer pole/1
  Set filer pole/1 -> Add2/2
  Filter gain for unity at 0 freq/1 -> Add2/1
  Add1/1 -> "[0,1] normalization unfiltered speed est from delta angle"/1, DeltaAngle/1

== system singleRotor_speedCTRL_dynInflow_PittPeters/Subsystem ==
  Rotor Speed (rad/s) : Inport
  Thrust : Inport  Port=2
  "Aero Power " : Scope
  Aero Torque : Sum
  Constant : Constant  Value=1.5
  Constant2 : Constant  Value=Cp0
  Gain2 : Gain  Gain=rho_air*(d_prop/2)^5*pi
  Gain4 : Gain  Gain=kappa/(rho_air*(d_prop/2)^2*pi)^.5/sqrt(2)
  Induced Torque : Product  Inputs=*/
  Power : Math  Operator=pow
  Product : Product
  Profile Torque : Product
  Qaero : Scope
  Square1 : Math  Operator=square
  To Workspace2 : ToWorkspace  VariableName=P_rotor  SaveFormat=Timeseries  SampleTime=-1
  Rotor Torque : Outport
  wires:
  Thrust/1 -> Power/1
  Square1/1 -> Profile Torque/1
  Aero Torque/1 -> Product/1, Rotor Torque/1, Qaero/1
  Gain2/1 -> Profile Torque/2
  Rotor Speed (rad/s)/1 -> Square1/1, Product/2, Induced Torque/2
  Induced Torque/1 -> Aero Torque/1
  Constant/1 -> Power/2
  Profile Torque/1 -> Aero Torque/2
  Power/1 -> Gain4/1
  Gain4/1 -> Induced Torque/1
  Constant2/1 -> Gain2/1
  Product/1 -> "Aero Power "/1, To Workspace2/1

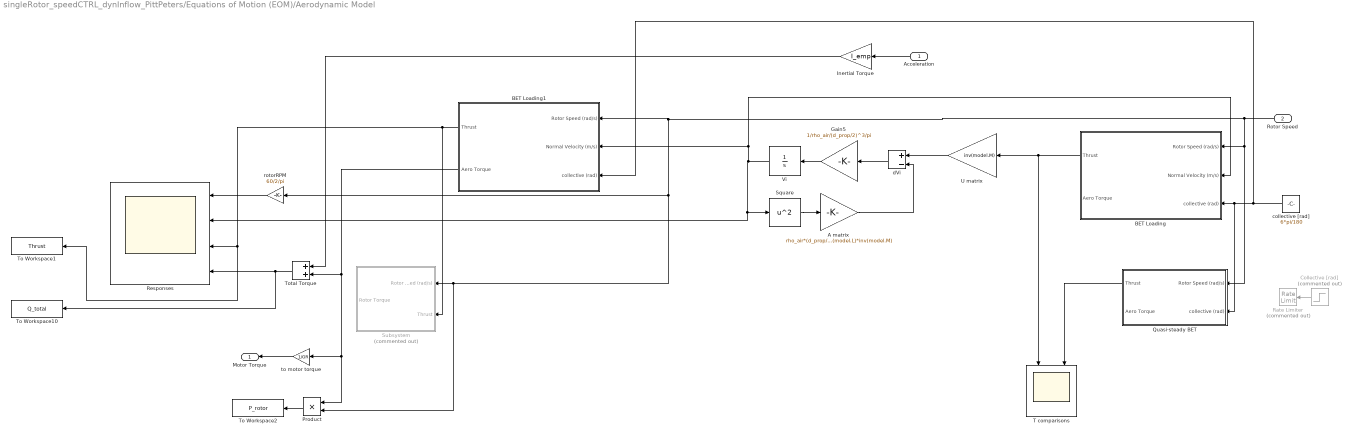
== system singleRotor_speedCTRL_dynInflow_PittPeters/Equations of Motion (EOM)/Aerodynamic Model ==
  Acceleration : Inport
  Rotor Speed : Inport  Port=2
  A matrix : Gain  Gain=rho_air*(d_prop/2)^2*pi*k*inv(model.L)*inv(model.M)
  BET Loading : Subsystem
  BET Loading1 : Subsystem
  Collective [rad] : Step  Commented=on  Time=8  Before=6*pi/180  After=5.65*pi/180  SampleTime=0
  Gain5 : Gain  Gain=1/rho_air/(d_prop/2)^3/pi
  Inertial Torque : Gain  Gain=I_emp
  Product : Product
  Quasi-steady BET : Subsystem
  Rate Limiter : RateLimiter  Commented=on  RisingSlewLimit=1.75*pi/180  FallingSlewLimit=-1.75*pi/180  SampleTimeMode=inherited
  Responses : Scope  NumInputPorts=4
  Square : Math  Operator=square
  Subsystem : Subsystem  Commented=on
  T comparisons : Scope  NumInputPorts=2
  To Workspace1 : ToWorkspace  VariableName=Thrust  SaveFormat=Timeseries  SampleTime=-1
  To Workspace10 : ToWorkspace  VariableName=Q_total  SaveFormat=Timeseries  SampleTime=-1
  To Workspace2 : ToWorkspace  VariableName=P_rotor  SaveFormat=Timeseries  SampleTime=-1
  Total Torque : Sum
  U matrix : Gain  Gain=inv(model.M)
  Vi : Integrator
  collective [rad] : Constant  Value=6*pi/180
  dVi : Sum  Inputs=+-
  rotorRPM : Gain  Gain=60/2/pi
  to motor torque : Gain  Gain=1/GR
  Motor Torque : Outport
  wires:
  Total Torque/1 -> To Workspace10/1, Responses/4
  Rotor Speed/1 -> BET Loading1/1(Rotor Speed (rad/s)), Subsystem/1(Rotor Speed (rad/s)), Product/2, rotorRPM/1, BET Loading/1(Rotor Speed (rad/s)), Quasi-steady BET/1(Rotor Speed (rad/s))
  Inertial Torque/1 -> Total Torque/1
  U matrix/1 -> dVi/1
  Acceleration/1 -> Inertial Torque/1
  Vi/1 -> BET Loading1/2(Normal Velocity (m/s)), BET Loading/2(Normal Velocity (m/s)), Responses/2, Square/1
  rotorRPM/1 -> Responses/1
  collective [rad]/1 -> BET Loading1/3(collective (rad)), Quasi-steady BET/2(collective (rad)), BET Loading/3(collective (rad))
  Gain5/1 -> Vi/1
  dVi/1 -> Gain5/1
  BET Loading/1(Thrust) -> T comparisons/1, U matrix/1
  Quasi-steady BET/1(Thrust) -> T comparisons/2
  Square/1 -> A matrix/1
  A matrix/1 -> dVi/2
  to motor torque/1 -> Motor Torque/1
  BET Loading1/1(Thrust) -> Subsystem/2(Thrust), To Workspace1/1, Responses/3
  BET Loading1/2(Aero Torque) -> Total Torque/2, Product/1, to motor torque/1
  Product/1 -> To Workspace2/1
  Collective [rad]/1 -> Rate Limiter/1

== system singleRotor_speedCTRL_dynInflow_PittPeters/Equations of Motion (EOM)/Transmission Model ==
  Accel_m : Inport
  Spd_m : Inport  Port=2
  Clock : Clock
  Clock1 : Clock
  Floor : Rounding
  Floor1 : Rounding
  Switch : Switch  Criteria=u2 > Threshold  SaturateOnIntegerOverflow=off  InputSameDT=off
  Switch1 : Switch  Criteria=u2 > Threshold  SaturateOnIntegerOverflow=off  InputSameDT=off
  to rotor accel : Gain  Gain=1/GR
  to rotor speed : Gain  Gain=1/GR
  transmission TF_tfest : TransferFcn  Numerator="[0\t0\t7145.76733952843]"  Denominator="[1\t12.0965895718261\t8502.35582966363]"
  transmission TF_tfest1 : TransferFcn  Numerator="[0\t0\t7145.76733952843]"  Denominator="[1\t12.0965895718261\t8502.35582966363]"
  Accel_r : Outport
  Spd_r : Outport  Port=2
  wires:
  Spd_m/1 -> transmission TF_tfest/1, to rotor speed/1
  Clock/1 -> Floor/1
  Floor/1 -> Switch/2
  to rotor speed/1 -> Spd_r/1, Switch/3
  transmission TF_tfest1/1 -> Switch1/1
  Floor1/1 -> Switch1/2
  Accel_m/1 -> to rotor accel/1, transmission TF_tfest1/1
  to rotor accel/1 -> Accel_r/1, Switch1/3
  Clock1/1 -> Floor1/1
  transmission TF_tfest/1 -> Switch/1

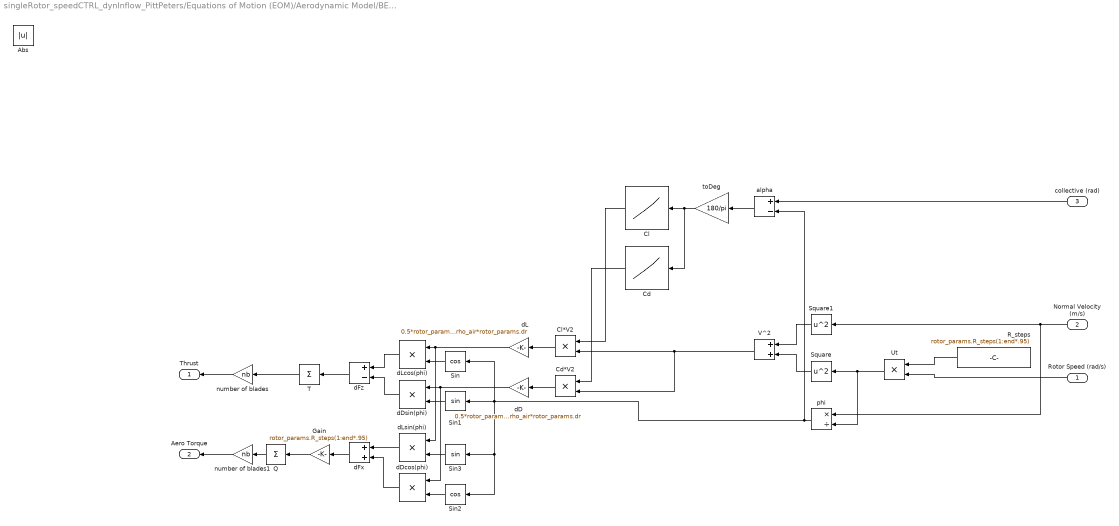
== system singleRotor_speedCTRL_dynInflow_PittPeters/Equations of Motion (EOM)/Aerodynamic Model/BET Loading ==
  Rotor Speed (rad/s) : Inport
  Normal Velocity (m/s) : Inport  Port=2
  collective (rad) : Inport  Port=3
  Abs : Abs  SaturateOnIntegerOverflow=off
  Cd : Lookup_n-D  NumberOfTableDimensions=1  BreakpointsForDimension1=rotor_params.AoA  BreakpointsForDimension2=[1:3]  Table=rotor_params.Cd  InternalRulePriority=Speed  RndMeth=Simplest
  Cd*V2 : Product
  Cl : Lookup_n-D  NumberOfTableDimensions=1  BreakpointsForDimension1=rotor_params.AoA  BreakpointsForDimension2=[1:3]  Table=rotor_params.Cl  UseLastTableValue=on  InternalRulePriority=Speed  RndMeth=Simplest
  Cl*V2 : Product
  Gain : Gain  Gain=rotor_params.R_steps(1:end*.95)
  Q : Sum  Inputs=+
  R_steps : Constant  Value=rotor_params.R_steps(1:end*.95)
  Sin : Trigonometry  Operator=cos
  Sin1 : Trigonometry
  Sin2 : Trigonometry  Operator=cos
  Sin3 : Trigonometry
  Square : Math  Operator=square
  Square1 : Math  Operator=square
  T : Sum  Inputs=+
  Ut : Product
  V^2 : Sum
  alpha : Sum  Inputs=+-
  dD : Gain  Gain=0.5*rotor_params.c*rho_air*rotor_params.dr
  dDcos(phi) : Product
  dDsin(phi) : Product
  dFx : Sum
  dFz : Sum  Inputs=+-
  dL : Gain  Gain=0.5*rotor_params.c*rho_air*rotor_params.dr
  dLcos(phi) : Product
  dLsin(phi) : Product
  number of blades : Gain  Gain=nb
  number of blades1 : Gain  Gain=nb
  phi : Product  Inputs=*/
  toDeg : Gain  Gain=180/pi
  Thrust : Outport
  Aero Torque : Outport  Port=2
  wires:
  T/1 -> number of blades/1
  alpha/1 -> toDeg/1
  Normal Velocity (m/s)/1 -> phi/1, Square1/1
  Rotor Speed (rad/s)/1 -> Ut/2
  phi/1 -> Sin/1, Sin1/1, Sin3/1, Sin2/1, alpha/2
  collective (rad)/1 -> alpha/1
  Square/1 -> V^2/2
  Square1/1 -> V^2/1
  Ut/1 -> phi/2, Square/1
  V^2/1 -> Cl*V2/2, Cd*V2/2
  R_steps/1 -> Ut/1
  Cl*V2/1 -> dL/1
  Cd*V2/1 -> dD/1
  Sin/1 -> dLcos(phi)/2
  dL/1 -> dLsin(phi)/1, dLcos(phi)/1
  dD/1 -> dDsin(phi)/1, dDcos(phi)/1
  Sin1/1 -> dDsin(phi)/2
  dLcos(phi)/1 -> dFz/1
  dDsin(phi)/1 -> dFz/2
  dFz/1 -> T/1
  number of blades/1 -> Thrust/1
  toDeg/1 -> Cl/1, Cd/1
  Cd/1 -> Cd*V2/1
  Q/1 -> number of blades1/1
  dFx/1 -> Gain/1
  Gain/1 -> Q/1
  Cl/1 -> Cl*V2/1
  Sin3/1 -> dLsin(phi)/2
  Sin2/1 -> dDcos(phi)/2
  dLsin(phi)/1 -> dFx/1
  dDcos(phi)/1 -> dFx/2
  number of blades1/1 -> Aero Torque/1

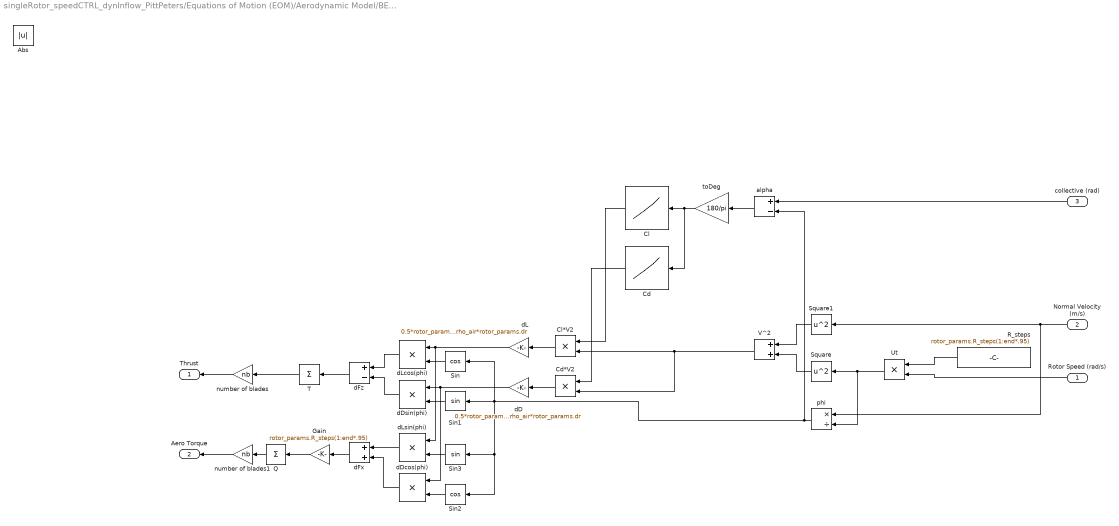
== system singleRotor_speedCTRL_dynInflow_PittPeters/Equations of Motion (EOM)/Aerodynamic Model/BET Loading1 ==
  Rotor Speed (rad/s) : Inport
  Normal Velocity (m/s) : Inport  Port=2
  collective (rad) : Inport  Port=3
  Abs : Abs  SaturateOnIntegerOverflow=off
  Cd : Lookup_n-D  NumberOfTableDimensions=1  BreakpointsForDimension1=rotor_params.AoA  BreakpointsForDimension2=[1:3]  Table=rotor_params.Cd  InternalRulePriority=Speed  RndMeth=Simplest
  Cd*V2 : Product
  Cl : Lookup_n-D  NumberOfTableDimensions=1  BreakpointsForDimension1=rotor_params.AoA  BreakpointsForDimension2=[1:3]  Table=rotor_params.Cl  UseLastTableValue=on  InternalRulePriority=Speed  RndMeth=Simplest
  Cl*V2 : Product
  Gain : Gain  Gain=rotor_params.R_steps(1:end*.95)
  Q : Sum  Inputs=+
  R_steps : Constant  Value=rotor_params.R_steps(1:end*.95)
  Sin : Trigonometry  Operator=cos
  Sin1 : Trigonometry
  Sin2 : Trigonometry  Operator=cos
  Sin3 : Trigonometry
  Square : Math  Operator=square
  Square1 : Math  Operator=square
  T : Sum  Inputs=+
  Ut : Product
  V^2 : Sum
  alpha : Sum  Inputs=+-
  dD : Gain  Gain=0.5*rotor_params.c*rho_air*rotor_params.dr
  dDcos(phi) : Product
  dDsin(phi) : Product
  dFx : Sum
  dFz : Sum  Inputs=+-
  dL : Gain  Gain=0.5*rotor_params.c*rho_air*rotor_params.dr
  dLcos(phi) : Product
  dLsin(phi) : Product
  number of blades : Gain  Gain=nb
  number of blades1 : Gain  Gain=nb
  phi : Product  Inputs=*/
  toDeg : Gain  Gain=180/pi
  Thrust : Outport
  Aero Torque : Outport  Port=2
  wires:
  T/1 -> number of blades/1
  alpha/1 -> toDeg/1
  Normal Velocity (m/s)/1 -> phi/1, Square1/1
  Rotor Speed (rad/s)/1 -> Ut/2
  phi/1 -> Sin/1, Sin1/1, Sin3/1, Sin2/1, alpha/2
  collective (rad)/1 -> alpha/1
  Square/1 -> V^2/2
  Square1/1 -> V^2/1
  Ut/1 -> phi/2, Square/1
  V^2/1 -> Cl*V2/2, Cd*V2/2
  R_steps/1 -> Ut/1
  Cl*V2/1 -> dL/1
  Cd*V2/1 -> dD/1
  Sin/1 -> dLcos(phi)/2
  dL/1 -> dLsin(phi)/1, dLcos(phi)/1
  dD/1 -> dDsin(phi)/1, dDcos(phi)/1
  Sin1/1 -> dDsin(phi)/2
  dLcos(phi)/1 -> dFz/1
  dDsin(phi)/1 -> dFz/2
  dFz/1 -> T/1
  number of blades/1 -> Thrust/1
  toDeg/1 -> Cl/1, Cd/1
  Cd/1 -> Cd*V2/1
  Q/1 -> number of blades1/1
  dFx/1 -> Gain/1
  Gain/1 -> Q/1
  Cl/1 -> Cl*V2/1
  Sin3/1 -> dLsin(phi)/2
  Sin2/1 -> dDcos(phi)/2
  dLsin(phi)/1 -> dFx/1
  dDcos(phi)/1 -> dFx/2
  number of blades1/1 -> Aero Torque/1

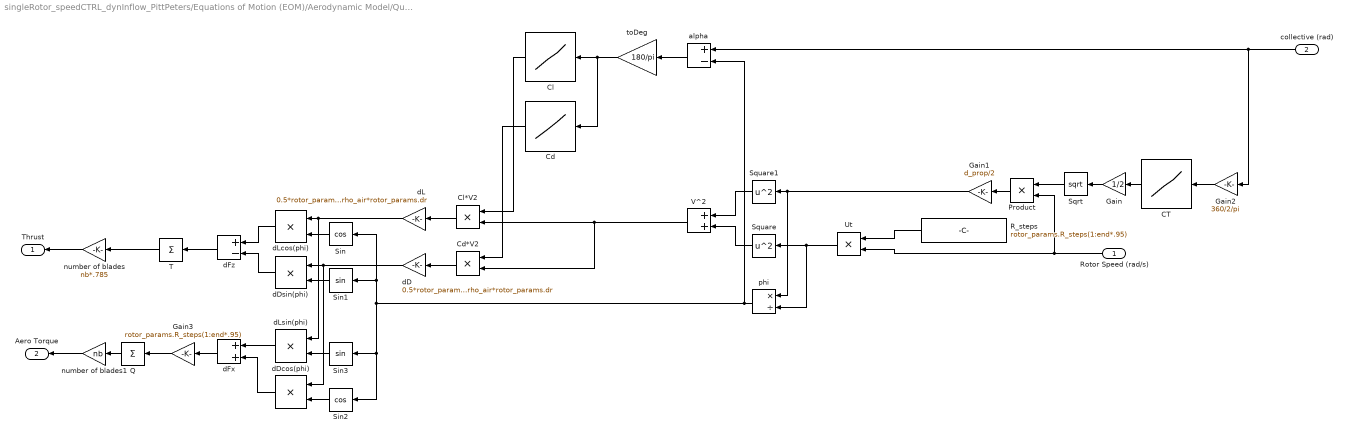
== system singleRotor_speedCTRL_dynInflow_PittPeters/Equations of Motion (EOM)/Aerodynamic Model/Quasi-steady BET ==
  Rotor Speed (rad/s) : Inport
  collective (rad) : Inport  Port=2
  CT : Lookup_n-D  NumberOfTableDimensions=1  BreakpointsForDimension1=theta  BreakpointsForDimension2=[1:3]  Table=Ct  UseLastTableValue=on  InternalRulePriority=Speed  RndMeth=Simplest
  Cd : Lookup_n-D  NumberOfTableDimensions=1  BreakpointsForDimension1=rotor_params.AoA  BreakpointsForDimension2=[1:3]  Table=rotor_params.Cd  InternalRulePriority=Speed  RndMeth=Simplest
  Cd*V2 : Product
  Cl : Lookup_n-D  NumberOfTableDimensions=1  BreakpointsForDimension1=rotor_params.AoA  BreakpointsForDimension2=[1:3]  Table=rotor_params.Cl  UseLastTableValue=on  InternalRulePriority=Speed  RndMeth=Simplest
  Cl*V2 : Product
  Gain : Gain  Gain=1/2
  Gain1 : Gain  Gain=d_prop/2
  Gain2 : Gain  Gain=360/2/pi
  Gain3 : Gain  Gain=rotor_params.R_steps(1:end*.95)
  Product : Product
  Q : Sum  Inputs=+
  R_steps : Constant  Value=rotor_params.R_steps(1:end*.95)
  Sin : Trigonometry  Operator=cos
  Sin1 : Trigonometry
  Sin2 : Trigonometry  Operator=cos
  Sin3 : Trigonometry
  Sqrt : Sqrt
  Square : Math  Operator=square
  Square1 : Math  Operator=square
  T : Sum  Inputs=+
  Ut : Product
  V^2 : Sum
  alpha : Sum  Inputs=+-
  dD : Gain  Gain=0.5*rotor_params.c*rho_air*rotor_params.dr
  dDcos(phi) : Product
  dDsin(phi) : Product
  dFx : Sum
  dFz : Sum  Inputs=+-
  dL : Gain  Gain=0.5*rotor_params.c*rho_air*rotor_params.dr
  dLcos(phi) : Product
  dLsin(phi) : Product
  number of blades : Gain  Gain=nb*.785
  number of blades1 : Gain  Gain=nb
  phi : Product  Inputs=*/
  toDeg : Gain  Gain=180/pi
  Thrust : Outport
  Aero Torque : Outport  Port=2
  wires:
  T/1 -> number of blades/1
  alpha/1 -> toDeg/1
  Rotor Speed (rad/s)/1 -> Product/2, Ut/2
  collective (rad)/1 -> Gain2/1, alpha/1
  Square/1 -> V^2/2
  Square1/1 -> V^2/1
  Ut/1 -> phi/2, Square/1
  V^2/1 -> Cl*V2/2, Cd*V2/2
  R_steps/1 -> Ut/1
  Cl*V2/1 -> dL/1
  Cd*V2/1 -> dD/1
  Sin/1 -> dLcos(phi)/2
  Sin1/1 -> dDsin(phi)/2
  dLcos(phi)/1 -> dFz/1
  dDsin(phi)/1 -> dFz/2
  dFz/1 -> T/1
  number of blades/1 -> Thrust/1
  toDeg/1 -> Cd/1, Cl/1
  Cl/1 -> Cl*V2/1
  Cd/1 -> Cd*V2/1
  CT/1 -> Gain/1
  Gain/1 -> Sqrt/1
  Sqrt/1 -> Product/1
  Product/1 -> Gain1/1
  Gain2/1 -> CT/1
  Gain1/1 -> phi/1, Square1/1
  phi/1 -> Sin/1, Sin1/1, Sin2/1, Sin3/1, alpha/2
  dL/1 -> dLcos(phi)/1, dLsin(phi)/1
  Q/1 -> number of blades1/1
  number of blades1/1 -> Aero Torque/1
  Sin2/1 -> dDcos(phi)/2
  dLsin(phi)/1 -> dFx/1
  dD/1 -> dDsin(phi)/1, dDcos(phi)/1
  dDcos(phi)/1 -> dFx/2
  Gain3/1 -> Q/1
  dFx/1 -> Gain3/1
  Sin3/1 -> dLsin(phi)/2

== system singleRotor_speedCTRL_dynInflow_PittPeters/Equations of Motion (EOM)/Aerodynamic Model/Subsystem ==
  Rotor Speed (rad/s) : Inport
  Thrust : Inport  Port=2
  "Aero Power " : Scope
  Aero Torque : Sum
  Constant : Constant  Value=1.5
  Constant2 : Constant  Value=Cp0
  Gain2 : Gain  Gain=rho_air*(d_prop/2)^5*pi
  Gain4 : Gain  Gain=kappa/(rho_air*(d_prop/2)^2*pi)^.5/sqrt(2)
  Induced Torque : Product  Inputs=*/
  Power : Math  Operator=pow
  Product : Product
  Profile Torque : Product
  Qaero : Scope
  Square1 : Math  Operator=square
  Rotor Torque : Outport
  wires:
  Thrust/1 -> Power/1
  Square1/1 -> Profile Torque/1
  Aero Torque/1 -> Product/1, Rotor Torque/1, Qaero/1
  Gain2/1 -> Profile Torque/2
  Rotor Speed (rad/s)/1 -> Square1/1, Product/2, Induced Torque/2
  Induced Torque/1 -> Aero Torque/1
  Constant/1 -> Power/2
  Profile Torque/1 -> Aero Torque/2
  Power/1 -> Gain4/1
  Gain4/1 -> Induced Torque/1
  Constant2/1 -> Gain2/1
  Product/1 -> "Aero Power "/1
